simulink model "Lab2"  (R2024b)
settings: Solver=FixedStepAuto  StartTime=0.0  StopTime=10.0  RelTol=1e-3  EnableMultiTasking=on
undefined symbols (not defined in the file): BOOL, DINT, OTL, slplc
libraries: simulink x8, arduinolib x3
(part 8 of 8)

== matlab function Lab2/PLC Controller Suite/__Logic/Task/Program/__Logic/XIC2/__Format ==
  data: BlockEnable input; RungIn input; RungOut input; data input
function setBlockFormat(BlockEnable, RungIn, RungOut, data)

if data~=0 && data~=1
    error('slplc:inivalidBooleanValue', 'Invalid boolean value %d', data);
end
data = logical(data);

% set parent block colors
coder.extrinsic('slplc.utils.setBlockAppearance');
persistent lastBlockEnable lastRungIn lastRungOut lastData isInit lastAnimation lastDataShow;
if isempty(lastBlockEnable)
    lastBlockEnable = true;
end
if isempty(lastRungIn)
    lastRungIn = false;
end
if isempty(lastRungOut)
    lastRungOut = false;
end
if isempty(lastData)
    lastData = data;
end
if isempty(isInit)
    isInit = true;
else
    isInit = false;
end
if isempty(lastAnimation)
    lastAnimation = false;
end
if isempty(lastDataShow)
    lastDataShow = false;
end

[animation, dataShow] = slplc.utils.setBlockAppearance('set', '%<PLCOperandTag>', {}, {}, ...
    ' = ', {'ForegroundColor'}, ...
    isInit,  ...
    BlockEnable, lastBlockEnable, ...
    RungIn,  lastRungIn, ...
    RungOut, lastRungOut, ...
    data, lastData, ...
    lastAnimation, lastDataShow);

lastBlockEnable = BlockEnable;
lastRungIn      = RungIn;
lastRungOut     = RungOut;
lastData        = data;
lastAnimation   = animation;
lastDataShow    = dataShow;
end

== matlab function Lab2/PLC Controller Suite/__Logic/Task/Program/__Logic/XIC5/__Format ==
  data: BlockEnable input; RungIn input; RungOut input; data input
function setBlockFormat(BlockEnable, RungIn, RungOut, data)

if data~=0 && data~=1
    error('slplc:inivalidBooleanValue', 'Invalid boolean value %d', data);
end
data = logical(data);

% set parent block colors
coder.extrinsic('slplc.utils.setBlockAppearance');
persistent lastBlockEnable lastRungIn lastRungOut lastData isInit lastAnimation lastDataShow;
if isempty(lastBlockEnable)
    lastBlockEnable = true;
end
if isempty(lastRungIn)
    lastRungIn = false;
end
if isempty(lastRungOut)
    lastRungOut = false;
end
if isempty(lastData)
    lastData = data;
end
if isempty(isInit)
    isInit = true;
else
    isInit = false;
end
if isempty(lastAnimation)
    lastAnimation = false;
end
if isempty(lastDataShow)
    lastDataShow = false;
end

[animation, dataShow] = slplc.utils.setBlockAppearance('set', '%<PLCOperandTag>', {}, {}, ...
    ' = ', {'ForegroundColor'}, ...
    isInit,  ...
    BlockEnable, lastBlockEnable, ...
    RungIn,  lastRungIn, ...
    RungOut, lastRungOut, ...
    data, lastData, ...
    lastAnimation, lastDataShow);

lastBlockEnable = BlockEnable;
lastRungIn      = RungIn;
lastRungOut     = RungOut;
lastData        = data;
lastAnimation   = animation;
lastDataShow    = dataShow;
end

== matlab function Lab2/PLC Controller Suite/__Logic/Task/Program/__Logic/XIO5/__Format ==
  data: BlockEnable input; RungIn input; RungOut input; data input
function setBlockFormat(BlockEnable, RungIn, RungOut, data)

if data~=0 && data~=1
    error('slplc:inivalidBooleanValue', 'Invalid boolean value %d', data);
end
data = logical(data);

% set parent block colors
coder.extrinsic('slplc.utils.setBlockAppearance');
persistent lastBlockEnable lastRungIn lastRungOut lastData isInit lastAnimation lastDataShow;
if isempty(lastBlockEnable)
    lastBlockEnable = true;
end
if isempty(lastRungIn)
    lastRungIn = false;
end
if isempty(lastRungOut)
    lastRungOut = false;
end
if isempty(lastData)
    lastData = data;
end
if isempty(isInit)
    isInit = true;
else
    isInit = false;
end
if isempty(lastAnimation)
    lastAnimation = false;
end
if isempty(lastDataShow)
    lastDataShow = false;
end

[animation, dataShow] = slplc.utils.setBlockAppearance('set', '%<PLCOperandTag>', {}, {}, ...
    ' = ', {'ForegroundColor'}, ...
    isInit,  ...
    BlockEnable, lastBlockEnable, ...
    RungIn,  lastRungIn, ...
    RungOut, lastRungOut, ...
    data, lastData, ...
    lastAnimation, lastDataShow);

lastBlockEnable = BlockEnable;
lastRungIn      = RungIn;
lastRungOut     = RungOut;
lastData        = data;
lastAnimation   = animation;
lastDataShow    = dataShow;
end

== matlab function Lab2/PLC Controller Suite/__Logic/Task/Program/__Logic/Junction4/__Format ==
  data: BlockEnable input; RungOut input
function setBlockFormat(BlockEnable, RungOut)
% set parent block colors
coder.extrinsic('slplc.utils.setBlockAppearance');
persistent lastBlockEnable isInit lastRungOut lastAnimation lastRungOutShow;
if isempty(lastBlockEnable)
    lastBlockEnable = true;
end

if isempty(isInit)
    isInit = true;
else
    isInit = false;
end

if isempty(lastRungOut)
    lastRungOut = RungOut;
end

if isempty(lastAnimation)
    lastAnimation = false;
end

if isempty(lastRungOutShow)
    lastRungOutShow = false;
end

[animation, dataShow] = slplc.utils.setBlockAppearance('set', '', {'black', 'black'}, {}, ...
    '', {'ForegroundColor', 'BackgroundColor'}, ...
    isInit,  ...
    BlockEnable, lastBlockEnable, ...
    RungOut,   lastRungOut, ...
    RungOut,   lastRungOut, ...
    [],    [], ...
    lastAnimation, lastRungOutShow);

lastBlockEnable     = BlockEnable;
lastRungOut         = RungOut;
lastAnimation       = animation;
lastRungOutShow     = dataShow;
end

== matlab function Lab2/PLC Controller Suite/__Logic/Task/Program/__Logic/Variable Read6/__Format ==
  data: data input
function setBlockFormat(data)
% set parent block colors
coder.extrinsic('slplc.utils.setBlockAppearance');
persistent isInit lastData  lastAnimation lastDataShow;

if isempty(isInit)
    isInit = true;
else
    isInit = false;
end

if isempty(lastData)
    lastData = data;
end

if isempty(lastAnimation)
    lastAnimation = false;
end

if isempty(lastDataShow)
    lastDataShow = false;
end

[animation, dataShow] = slplc.utils.setBlockAppearance('set', '', {}, {}, ...
    '%<PLCOperandTag> = ', {}, ...
    isInit,  ...
    true,  true, ...
    false, false, ...
    false, false, ...
    data,  lastData, ...
    lastAnimation, lastDataShow);

lastData        = data;
lastAnimation   = animation;
lastDataShow    = dataShow;
end

== matlab function Lab2/PLC Controller Suite/__Logic/Task/Program/__Logic/AND/__Format ==
  data: BlockEnable input; RungIn input; RungOut input
function setBlockFormat(BlockEnable, RungIn, RungOut)
% set parent block colors
coder.extrinsic('slplc.utils.setBlockAppearance');
persistent lastBlockEnable lastRungIn lastRungOut isInit lastAnimation lastDataShow;
if isempty(lastBlockEnable)
    lastBlockEnable = true;
end
if isempty(lastRungIn)
    lastRungIn = false;
end
if isempty(lastRungOut)
    lastRungOut = false;
end

if isempty(isInit)
    isInit = true;
else
    isInit = false;
end
if isempty(lastAnimation)
    lastAnimation = false;
end
if isempty(lastDataShow)
    lastDataShow = false;
end

[animation, dataShow] = slplc.utils.setBlockAppearance('set', '', {}, {}, ...
    ' = ',  {'ForegroundColor'}, ...
    isInit,  ...
    BlockEnable, lastBlockEnable, ...
    RungIn,  lastRungIn, ...
    RungOut, lastRungOut, ...
    [],    [], ...
    lastAnimation, lastDataShow);

lastBlockEnable = BlockEnable;
lastRungIn      = RungIn;
lastRungOut     = RungOut;
lastAnimation   = animation;
lastDataShow    = dataShow;
end

== matlab function Lab2/PLC Controller Suite/__Logic/Task/Program/__Logic/OR/__Format ==
  data: BlockEnable input; RungIn input; RungOut input
function setBlockFormat(BlockEnable, RungIn, RungOut)
% set parent block colors
coder.extrinsic('slplc.utils.setBlockAppearance');
persistent lastBlockEnable lastRungIn lastRungOut isInit lastAnimation lastDataShow;
if isempty(lastBlockEnable)
    lastBlockEnable = true;
end
if isempty(lastRungIn)
    lastRungIn = false;
end
if isempty(lastRungOut)
    lastRungOut = false;
end

if isempty(isInit)
    isInit = true;
else
    isInit = false;
end
if isempty(lastAnimation)
    lastAnimation = false;
end
if isempty(lastDataShow)
    lastDataShow = false;
end

[animation, dataShow] = slplc.utils.setBlockAppearance('set', '', {}, {}, ...
    ' = ',  {'ForegroundColor'}, ...
    isInit,  ...
    BlockEnable, lastBlockEnable, ...
    RungIn,  lastRungIn, ...
    RungOut, lastRungOut, ...
    [],    [], ...
    lastAnimation, lastDataShow);

lastBlockEnable = BlockEnable;
lastRungIn      = RungIn;
lastRungOut     = RungOut;
lastAnimation   = animation;
lastDataShow    = dataShow;
end

== matlab function Lab2/PLC Controller Suite/__Logic/Task/Program/__Logic/NOT/__Format ==
  data: BlockEnable input; RungIn input; RungOut input
function setBlockFormat(BlockEnable, RungIn, RungOut)
% set parent block colors
coder.extrinsic('slplc.utils.setBlockAppearance');
persistent lastBlockEnable lastRungIn lastRungOut isInit lastAnimation lastDataShow;
if isempty(lastBlockEnable)
    lastBlockEnable = true;
end
if isempty(lastRungIn)
    lastRungIn = false;
end
if isempty(lastRungOut)
    lastRungOut = false;
end

if isempty(isInit)
    isInit = true;
else
    isInit = false;
end
if isempty(lastAnimation)
    lastAnimation = false;
end
if isempty(lastDataShow)
    lastDataShow = false;
end

[animation, dataShow] = slplc.utils.setBlockAppearance('set', '', {}, {}, ...
    ' = ',  {'ForegroundColor'}, ...
    isInit,  ...
    BlockEnable, lastBlockEnable, ...
    RungIn,  lastRungIn, ...
    RungOut, lastRungOut, ...
    [],    [], ...
    lastAnimation, lastDataShow);

lastBlockEnable = BlockEnable;
lastRungIn      = RungIn;
lastRungOut     = RungOut;
lastAnimation   = animation;
lastDataShow    = dataShow;
end

== matlab function Lab2/PLC Controller Suite/__Logic/Task/Program/__Logic/LES/__Format ==
  data: BlockEnable input; RungIn input; RungOut input
function setBlockFormat(BlockEnable, RungIn, RungOut)
% set parent block colors
coder.extrinsic('slplc.utils.setBlockAppearance');
persistent lastBlockEnable lastRungIn lastRungOut isInit lastAnimation lastDataShow;
if isempty(lastBlockEnable)
    lastBlockEnable = true;
end
if isempty(lastRungIn)
    lastRungIn = false;
end
if isempty(lastRungOut)
    lastRungOut = false;
end

if isempty(isInit)
    isInit = true;
else
    isInit = false;
end
if isempty(lastAnimation)
    lastAnimation = false;
end
if isempty(lastDataShow)
    lastDataShow = false;
end

[animation, dataShow] = slplc.utils.setBlockAppearance('set', '', {}, {}, ...
    ' = ',  {'ForegroundColor'}, ...
    isInit,  ...
    BlockEnable, lastBlockEnable, ...
    RungIn,  lastRungIn, ...
    RungOut, lastRungOut, ...
    [],    [], ...
    lastAnimation, lastDataShow);

lastBlockEnable = BlockEnable;
lastRungIn      = RungIn;
lastRungOut     = RungOut;
lastAnimation   = animation;
lastDataShow    = dataShow;
end

== matlab function Lab2/PLC Controller Suite/__Logic/Task/Program/__Logic/Power Rail Start/__Format ==
  data: RungOut input
function setBlockFormat(RungOut)
% set parent block colors
coder.extrinsic('slplc.utils.setBlockAppearance');
persistent isInit lastRungOut lastAnimation lastRungOutShow;

if isempty(isInit)
    isInit = true;
else
    isInit = false;
end

if isempty(lastRungOut)
    lastRungOut = RungOut;
end

if isempty(lastAnimation)
    lastAnimation = false;
end

if isempty(lastRungOutShow)
    lastRungOutShow = false;
end

[animation, dataShow] = slplc.utils.setBlockAppearance('set', '', {'black', 'black'}, {}, ...
    '', {'ForegroundColor', 'BackgroundColor'}, ...
    isInit,  ...
    true,  true, ...
    RungOut,   lastRungOut, ...
    RungOut,   lastRungOut, ...
    [],    [], ...
    lastAnimation, lastRungOutShow);

lastRungOut         = RungOut;
lastAnimation       = animation;
lastRungOutShow     = dataShow;
end

== matlab function Lab2/PLC Controller Suite/__Logic/Task/Program/__Logic/AND/Instruction_Enable/type_process2 ==
  data: u input size=1; y output int32 size=1
function y = typeProcess(u)

if isa(u, 'int8')
    % SINT
    if u<0
        y = int32(256) + int32(u);
    else
        y = int32(u);
    end
elseif isa(u, 'int16')
    % INT                
    if u < 0
        y = int32(65536) + int32(u);
    else
        y = int32(u);
    end
elseif isa(u, 'int32')
    % DINT
    y = u;    
elseif isa(u, 'single') || isa(u, 'double')
    % REAL
    y = int32(convergent(u));    
else
    % Invalid Data Type
    error('slplc:invalidDataType', ...
        'Invalid source data type %s for bitwise instruction block', ...
        class(u));
end

end

== matlab function Lab2/PLC Controller Suite/__Logic/Task/Program/__Logic/OR/Instruction_Enable/type_process1 ==
  data: u input size=1; y output int32 size=1
function y = typeProcess(u)

if isa(u, 'int8')
    % SINT
    if u<0
        y = int32(256) + int32(u);
    else
        y = int32(u);
    end
elseif isa(u, 'int16')
    % INT                
    if u < 0
        y = int32(65536) + int32(u);
    else
        y = int32(u);
    end
elseif isa(u, 'int32')
    % DINT
    y = u;    
elseif isa(u, 'single') || isa(u, 'double')
    % REAL
    y = int32(convergent(u));    
else
    % Invalid Data Type
    error('slplc:invalidDataType', ...
        'Invalid source data type %s for bitwise instruction block', ...
        class(u));
end

end

== matlab function Lab2/PLC Controller Suite/__Logic/Task/Program/__Logic/OR/Instruction_Enable/type_process2 ==
  data: u input size=1; y output int32 size=1
function y = typeProcess(u)

if isa(u, 'int8')
    % SINT
    if u<0
        y = int32(256) + int32(u);
    else
        y = int32(u);
    end
elseif isa(u, 'int16')
    % INT                
    if u < 0
        y = int32(65536) + int32(u);
    else
        y = int32(u);
    end
elseif isa(u, 'int32')
    % DINT
    y = u;    
elseif isa(u, 'single') || isa(u, 'double')
    % REAL
    y = int32(convergent(u));    
else
    % Invalid Data Type
    error('slplc:invalidDataType', ...
        'Invalid source data type %s for bitwise instruction block', ...
        class(u));
end

end

== matlab function Lab2/PLC Controller Suite/__Logic/Task/Program/__Logic/Variable Read5/__Format ==
  data: data input
function setBlockFormat(data)
% set parent block colors
coder.extrinsic('slplc.utils.setBlockAppearance');
persistent isInit lastData  lastAnimation lastDataShow;

if isempty(isInit)
    isInit = true;
else
    isInit = false;
end

if isempty(lastData)
    lastData = data;
end

if isempty(lastAnimation)
    lastAnimation = false;
end

if isempty(lastDataShow)
    lastDataShow = false;
end

[animation, dataShow] = slplc.utils.setBlockAppearance('set', '', {}, {}, ...
    '%<PLCOperandTag> = ', {}, ...
    isInit,  ...
    true,  true, ...
    false, false, ...
    false, false, ...
    data,  lastData, ...
    lastAnimation, lastDataShow);

lastData        = data;
lastAnimation   = animation;
lastDataShow    = dataShow;
end

== matlab function Lab2/PLC Controller Suite/__Logic/Task/Program/__Logic/NOT/Instruction_Enable/type_process1 ==
  data: u input size=1; y output int32 size=1
function y = typeProcess(u)

if isa(u, 'int8')
    % SINT
    if u<0
        y = int32(256) + int32(u);
    else
        y = int32(u);
    end
elseif isa(u, 'int16')
    % INT                
    if u < 0
        y = int32(65536) + int32(u);
    else
        y = int32(u);
    end
elseif isa(u, 'int32')
    % DINT
    y = u;    
elseif isa(u, 'single') || isa(u, 'double')
    % REAL
    y = int32(convergent(u));    
else
    % Invalid Data Type
    error('slplc:invalidDataType', ...
        'Invalid source data type %s for bitwise instruction block', ...
        class(u));
end

end

== matlab function Lab2/PLC Controller Suite/__Logic/Task/Program/__Logic/OTL/__Format ==
  data: BlockEnable input; RungIn input; RungOut input; data input
function setBlockFormat(BlockEnable, RungIn, RungOut, data)

if data~=0 && data~=1
    error('slplc:inivalidBooleanValue', 'Invalid boolean value %d', data);
end
data = logical(data);

% set parent block colors
coder.extrinsic('slplc.utils.setBlockAppearance');
persistent lastBlockEnable lastRungIn lastRungOut lastData isInit lastAnimation lastDataShow;
if isempty(lastBlockEnable)
    lastBlockEnable = true;
end
if isempty(lastRungIn)
    lastRungIn = false;
end
if isempty(lastRungOut)
    lastRungOut = false;
end
if isempty(lastData)
    lastData = data;
end
if isempty(isInit)
    isInit = true;
else
    isInit = false;
end
if isempty(lastAnimation)
    lastAnimation = false;
end
if isempty(lastDataShow)
    lastDataShow = false;
end

[animation, dataShow] = slplc.utils.setBlockAppearance('set', '%<PLCOperandTag>', {}, {}, ...
    ' = ', {'ForegroundColor'}, ...
    isInit,  ...
    BlockEnable, lastBlockEnable, ...
    RungIn,  lastRungIn, ...
    RungOut, lastRungOut, ...
    data, lastData, ...
    lastAnimation, lastDataShow);

lastBlockEnable = BlockEnable;
lastRungIn      = RungIn;
lastRungOut     = RungOut;
lastData        = data;
lastAnimation   = animation;
lastDataShow    = dataShow;
end

== matlab function Lab2/PLC Controller Suite/__Logic/Task/Program/__Logic/LES1/__Format ==
  data: BlockEnable input; RungIn input; RungOut input
function setBlockFormat(BlockEnable, RungIn, RungOut)
% set parent block colors
coder.extrinsic('slplc.utils.setBlockAppearance');
persistent lastBlockEnable lastRungIn lastRungOut isInit lastAnimation lastDataShow;
if isempty(lastBlockEnable)
    lastBlockEnable = true;
end
if isempty(lastRungIn)
    lastRungIn = false;
end
if isempty(lastRungOut)
    lastRungOut = false;
end

if isempty(isInit)
    isInit = true;
else
    isInit = false;
end
if isempty(lastAnimation)
    lastAnimation = false;
end
if isempty(lastDataShow)
    lastDataShow = false;
end

[animation, dataShow] = slplc.utils.setBlockAppearance('set', '', {}, {}, ...
    ' = ',  {'ForegroundColor'}, ...
    isInit,  ...
    BlockEnable, lastBlockEnable, ...
    RungIn,  lastRungIn, ...
    RungOut, lastRungOut, ...
    [],    [], ...
    lastAnimation, lastDataShow);

lastBlockEnable = BlockEnable;
lastRungIn      = RungIn;
lastRungOut     = RungOut;
lastAnimation   = animation;
lastDataShow    = dataShow;
end

== matlab function Lab2/PLC Controller Suite/__Logic/Task/Program/__Logic/Variable Read1/__Format ==
  data: data input
function setBlockFormat(data)
% set parent block colors
coder.extrinsic('slplc.utils.setBlockAppearance');
persistent isInit lastData  lastAnimation lastDataShow;

if isempty(isInit)
    isInit = true;
else
    isInit = false;
end

if isempty(lastData)
    lastData = data;
end

if isempty(lastAnimation)
    lastAnimation = false;
end

if isempty(lastDataShow)
    lastDataShow = false;
end

[animation, dataShow] = slplc.utils.setBlockAppearance('set', '', {}, {}, ...
    '%<PLCOperandTag> = ', {}, ...
    isInit,  ...
    true,  true, ...
    false, false, ...
    false, false, ...
    data,  lastData, ...
    lastAnimation, lastDataShow);

lastData        = data;
lastAnimation   = animation;
lastDataShow    = dataShow;
end

== matlab function Lab2/PLC Controller Suite/__Logic/Task/Program/__Logic/OTU/__Format ==
  data: BlockEnable input; RungIn input; RungOut input; data input
function setBlockFormat(BlockEnable, RungIn, RungOut, data)

if data~=0 && data~=1
    error('slplc:inivalidBooleanValue', 'Invalid boolean value %d', data);
end
data = logical(data);

% set parent block colors
coder.extrinsic('slplc.utils.setBlockAppearance');
persistent lastBlockEnable lastRungIn lastRungOut lastData isInit lastAnimation lastDataShow;
if isempty(lastBlockEnable)
    lastBlockEnable = true;
end
if isempty(lastRungIn)
    lastRungIn = false;
end
if isempty(lastRungOut)
    lastRungOut = false;
end
if isempty(lastData)
    lastData = data;
end
if isempty(isInit)
    isInit = true;
else
    isInit = false;
end
if isempty(lastAnimation)
    lastAnimation = false;
end
if isempty(lastDataShow)
    lastDataShow = false;
end

[animation, dataShow] = slplc.utils.setBlockAppearance('set', '%<PLCOperandTag>', {}, {}, ...
    ' = ', {'ForegroundColor'}, ...
    isInit,  ...
    BlockEnable, lastBlockEnable, ...
    RungIn,  lastRungIn, ...
    RungOut, lastRungOut, ...
    data, lastData, ...
    lastAnimation, lastDataShow);

lastBlockEnable = BlockEnable;
lastRungIn      = RungIn;
lastRungOut     = RungOut;
lastData        = data;
lastAnimation   = animation;
lastDataShow    = dataShow;
end

== matlab function Lab2/PLC Controller Suite/__Logic/Task/Program/__Logic/Junction/__Format ==
  data: BlockEnable input; RungOut input
function setBlockFormat(BlockEnable, RungOut)
% set parent block colors
coder.extrinsic('slplc.utils.setBlockAppearance');
persistent lastBlockEnable isInit lastRungOut lastAnimation lastRungOutShow;
if isempty(lastBlockEnable)
    lastBlockEnable = true;
end

if isempty(isInit)
    isInit = true;
else
    isInit = false;
end

if isempty(lastRungOut)
    lastRungOut = RungOut;
end

if isempty(lastAnimation)
    lastAnimation = false;
end

if isempty(lastRungOutShow)
    lastRungOutShow = false;
end

[animation, dataShow] = slplc.utils.setBlockAppearance('set', '', {'black', 'black'}, {}, ...
    '', {'ForegroundColor', 'BackgroundColor'}, ...
    isInit,  ...
    BlockEnable, lastBlockEnable, ...
    RungOut,   lastRungOut, ...
    RungOut,   lastRungOut, ...
    [],    [], ...
    lastAnimation, lastRungOutShow);

lastBlockEnable     = BlockEnable;
lastRungOut         = RungOut;
lastAnimation       = animation;
lastRungOutShow     = dataShow;
end

== matlab function Lab2/PLC Controller Suite/__Logic/Task/Program/__Logic/LES4/__Format ==
  data: BlockEnable input; RungIn input; RungOut input
function setBlockFormat(BlockEnable, RungIn, RungOut)
% set parent block colors
coder.extrinsic('slplc.utils.setBlockAppearance');
persistent lastBlockEnable lastRungIn lastRungOut isInit lastAnimation lastDataShow;
if isempty(lastBlockEnable)
    lastBlockEnable = true;
end
if isempty(lastRungIn)
    lastRungIn = false;
end
if isempty(lastRungOut)
    lastRungOut = false;
end

if isempty(isInit)
    isInit = true;
else
    isInit = false;
end
if isempty(lastAnimation)
    lastAnimation = false;
end
if isempty(lastDataShow)
    lastDataShow = false;
end

[animation, dataShow] = slplc.utils.setBlockAppearance('set', '', {}, {}, ...
    ' = ',  {'ForegroundColor'}, ...
    isInit,  ...
    BlockEnable, lastBlockEnable, ...
    RungIn,  lastRungIn, ...
    RungOut, lastRungOut, ...
    [],    [], ...
    lastAnimation, lastDataShow);

lastBlockEnable = BlockEnable;
lastRungIn      = RungIn;
lastRungOut     = RungOut;
lastAnimation   = animation;
lastDataShow    = dataShow;
end
